simulink model "costas_loop"  (R2013a)
settings: Solver=ode3  StartTime=0.0  StopTime=5/1200  FixedStep=1/120000  RelTol=1e-3
libraries: dsparch4 x6, commsynccomp2 x2, commrandsrc2 x1, commsink2 x1, commfilt2 x1
settings Model: Creator=tibbs2010  LastModifiedBy=tibbs2010

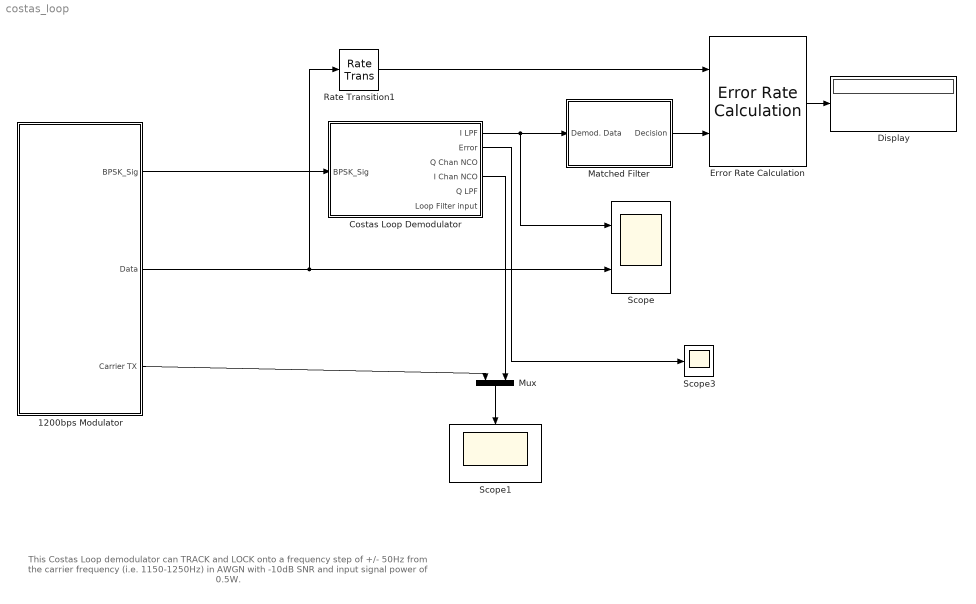
== system costas_loop ==
  note: This Costas Loop demodulator can TRACK and LOCK onto a
      |  frequency step of +/- 50Hz from the carrier frequency (i.e. 1150-1250Hz)
      | in AWGN with -10dB SNR and input signal power of 0.5W.
  1200bps Modulator : Subsystem
  Costas Loop Demodulator : Subsystem
  Display : Display
  Error Rate Calculation : commsink2/Error Rate Calculation  N=1  st_delay=0  cp_mode=Entire frame  subframe=[]  PMode=Port  WsName=ErrorVec  RsMode2=off  stop=off  numErr=100  maxBits=1e6
  Matched Filter : Subsystem
  Mux : Mux  Inputs=2
  Rate Transition1 : RateTransition  OutPortSampleTime=1/1200
  Scope : Scope  NumInputPorts=2
      settings: YMin=-0.3~-2  YMax=0.3~2
  Scope1 : Scope
      settings: YMin=-0.3  YMax=0.3
  Scope3 : Scope
      settings: YMin=-1  YMax=1  SaveName=ScopeData3
  wires:
  Costas Loop Demodulator/1(I LPF) -> Matched Filter/1(Demod. Data), Scope/1
  Error Rate Calculation/1 -> Display/1
  Mux/1 -> Scope1/1
  1200bps Modulator/3(Carrier TX) -> Mux/1
  Costas Loop Demodulator/4(I Chan NCO) -> Mux/2
  Costas Loop Demodulator/2(Error) -> Scope3/1
  1200bps Modulator/2(Data) -> Rate Transition1/1, Scope/2
  Rate Transition1/1 -> Error Rate Calculation/1
  Matched Filter/1(Decision) -> Error Rate Calculation/2
  1200bps Modulator/1(BPSK_Sig) -> Costas Loop Demodulator/1(BPSK_Sig)

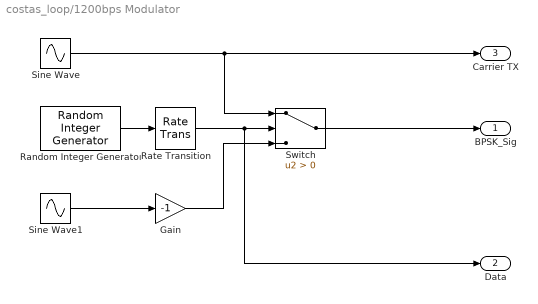
== system costas_loop/1200bps Modulator ==
  Gain : Gain  Gain=-1
  Random Integer Generator : commrandsrc2/Random Integer Generator  mul=2  seed=randseed  Ts=1/1200  frameBased=off  sampPerFrame=1  orient=off  outDataType=double
  Rate Transition : RateTransition  OutPortSampleTime=1/120000
  Sine Wave : Sin  Frequency=2*pi*10e3  Phase=pi/2  Samples=1024  SampleTime=1/120000
  Sine Wave1 : Sin  Frequency=2*pi*10e3  Phase=pi/2  Samples=1024  SampleTime=1/120000
  Switch : Switch  Criteria=u2 > Threshold
  BPSK_Sig : Outport
  Data : Outport  Port=2
  Carrier TX : Outport  Port=3
  wires:
  Random Integer Generator/1 -> Rate Transition/1
  Rate Transition/1 -> Data/1, Switch/2
  Sine Wave/1 -> Carrier TX/1, Switch/1
  Sine Wave1/1 -> Gain/1
  Gain/1 -> Switch/3
  Switch/1 -> BPSK_Sig/1

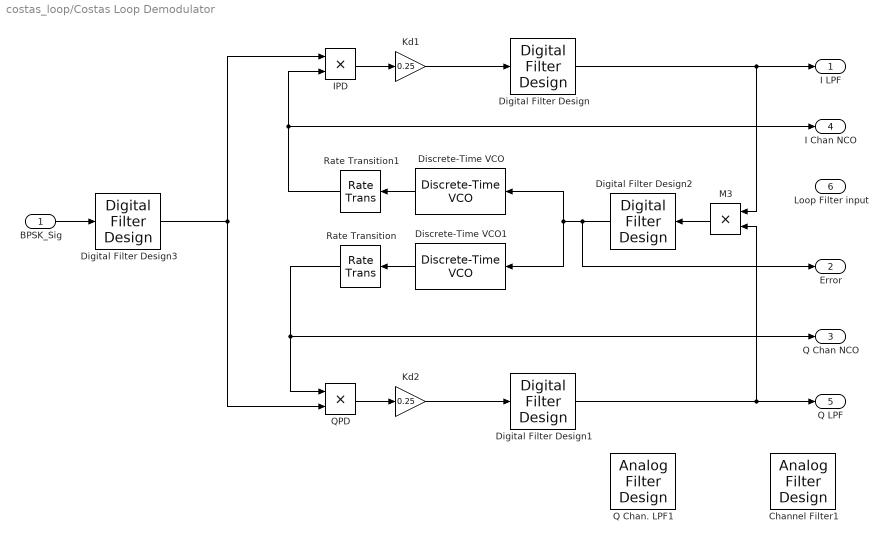
== system costas_loop/Costas Loop Demodulator ==
  BPSK_Sig : Inport
  Channel Filter1 : dsparch4/Analog Filter Design  method=Butterworth  filttype=Bandpass  N=2  Wlo=2*pi*600  Whi=2*pi*2400  Rp=2  Rs=40
  Digital Filter Design{,1..3} (4 alike) : dsparch4/Digital Filter Design  mwdsp_browser_bugfix_var=off
  Discrete-Time VCO : commsynccomp2/Discrete-Time VCO  Ac=1  Fc=10e3  Kc=2*10e3*8  Ph=0  ts=1/120000
  Discrete-Time VCO1 : commsynccomp2/Discrete-Time VCO  Ac=1  Fc=10e3  Kc=2*10e3*8  Ph=pi/2  ts=1/120000
  IPD : Product
  Kd1 : Gain  Gain=0.25
  Kd2 : Gain  Gain=0.25
  M3 : Product
  Q Chan. LPF1 : dsparch4/Analog Filter Design  method=Butterworth  filttype=Lowpass  N=1  Wlo=2*pi*2400  Whi=80  Rp=2  Rs=40
  QPD : Product
  Rate Transition : RateTransition  OutPortSampleTime=1/120000
  Rate Transition1 : RateTransition  OutPortSampleTime=1/120000
  I LPF : Outport
  Error : Outport  Port=2
  Q Chan NCO : Outport  Port=3
  I Chan NCO : Outport  Port=4
  Q LPF : Outport  Port=5
  Loop Filter input : Outport  Port=6
  wires:
  QPD/1 -> Kd2/1
  IPD/1 -> Kd1/1
  Discrete-Time VCO/1 -> Rate Transition1/1
  Discrete-Time VCO1/1 -> Rate Transition/1
  Digital Filter Design1/1 -> Q LPF/1, M3/2
  Kd2/1 -> Digital Filter Design1/1
  Rate Transition/1 -> QPD/1, Q Chan NCO/1
  Rate Transition1/1 -> IPD/2, I Chan NCO/1
  Kd1/1 -> Digital Filter Design/1
  Digital Filter Design/1 -> I LPF/1, M3/1
  M3/1 -> Digital Filter Design2/1
  BPSK_Sig/1 -> Digital Filter Design3/1
  Digital Filter Design2/1 -> Error/1, Discrete-Time VCO1/1, Discrete-Time VCO/1
  Digital Filter Design3/1 -> IPD/1, QPD/2

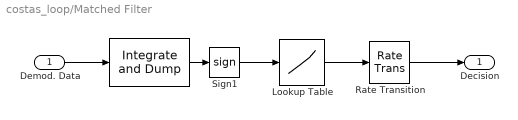
== system costas_loop/Matched Filter ==
  Demod. Data : Inport
  " " : commfilt2/Integrate and Dump  obssamples=10  offsetsamples=0  nodump=off  roundingMode=Floor  overflowMode=off
  Lookup Table : Lookup  InputValues=[-1,0,1]  Table=[0,0,1]
  Rate Transition : RateTransition  OutPortSampleTime=1/1200
  Sign1 : Signum
  Decision : Outport
  wires:
  Demod. Data/1 -> " "/1
  Sign1/1 -> Lookup Table/1
  Rate Transition/1 -> Decision/1
  " "/1 -> Sign1/1
  Lookup Table/1 -> Rate Transition/1
